simulink model "modechanger"  (R2022b)
settings: Solver=FixedStepAuto  StartTime=0.0  StopTime=inf  FixedStep=0.01  RelTol=1e-3
libraries: robotlib x7
settings Model: Creator=sprinkle  LastModifiedBy=sprinkle
settings SolverCC: AlgebraicLoopSolver=TrustRegion
settings OptimizationCC: UseFloatMulNetSlope=on  EnhancedBackFolding=on  EfficientFloat2IntCast=on  MaxStackSize=64  OptimizeBlockOrder=speed  DifferentSizesBufferReuse=on  OptimizationCustomize=off
settings DebuggingCC: ParameterTunabilityLossMsg=error  UnconnectedInputMsg=warning  UnconnectedOutputMsg=warning  UnconnectedLineMsg=warning  SFMachineParentedDataDiag=warning
settings HardwareCC: ProdBitPerPointer=32  ProdBitPerSizeT=32  ProdBitPerPtrDiffT=32  ProdLargestAtomicFloat=None  ProdIntDivRoundTo=Undefined  ProdEndianess=Unspecified  ProdWordSize=32  ProdHWDeviceType=Generic->Unspecified (assume 32-bit Generic)  UseEmbeddedCoderFeatures=off
settings ModelReferenceCC: EnableRefExpFcnMdlSchedulingChecks=on
settings SFSimCC: MATLABDynamicMemAlloc=off  SimTargetLang=C++
settings RTWCC: Description=Embedded Coder  SystemTargetFile=ert.tlc  HardwareBoard=Robot Operating System (ROS)  TLCOptions="-aInlineSetEventsForThisBaseRateFcn=TLC_FALSE -aSuppressMultiTaskScheduler=TLC_FALSE  -aRateBasedStepFcn=0"  TemplateMakefile=ert_default_tmf  GenerateReport=on  Toolchain=Catkin  BuildConfiguration=Faster Runs  LaunchReport=on  TargetLang=C++
settings CodeAppCC: ForceParamTrailComments=on  OperatorAnnotations=on
settings ERTTargetCC: ERTCustomFileBanners=off  SupportNonFinite=off  SupportContinuousTime=on  SupportNonInlinedSFcns=on  RemoveResetFunc=off  ModelStepFunctionPrototypeControlCompliant=off  RootIOFormat=Structure reference

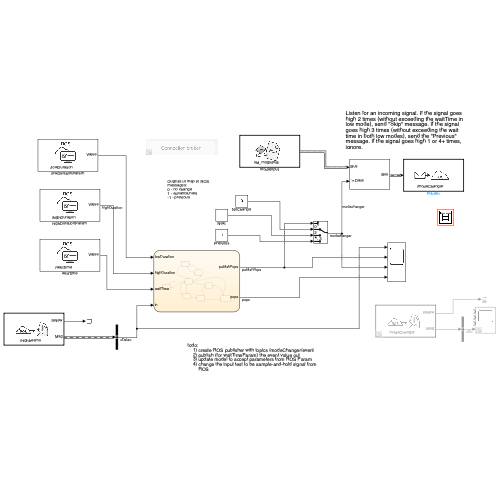
[thumbnail: Simulink's stored preview of the top-level diagram]
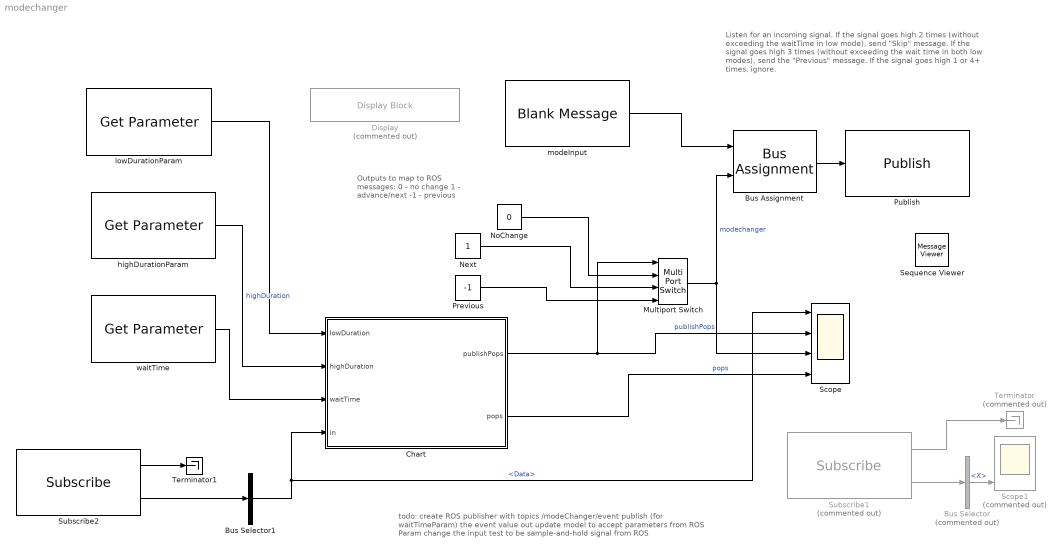
== system modechanger ==
  note: todo:
      | create ROS publisher with topics /modeChanger/event
      | publish (for waitTimeParam) the event value out
      | update model to accept parameters from ROS Param
      | change the input test to be sample-and-hold signal from ROS
  note: Listen for an incoming signal. If the signal goes high 2 times (without exceeding the waitTime in low mode), send "Skip" message. If the signal goes high 3 times (without exceeding the wait time in both low modes), send the "Previous" message. If the signal goes high 1 or 4+ times, ignore.
  note: Outputs to map to ROS messages:
      | 0 - no change
      | 1 - advance/next
      | -1 - previous
  Bus Assignment : BusAssignment  AssignedSignals=Data
  Bus Selector : BusSelector  Commented=on  DialogController=Simulink.DDGSource_BusSelector  OutputSignals=Linear.X
  Bus Selector1 : BusSelector  DialogController=Simulink.DDGSource_BusSelector  OutputSignals=Data
  Chart : Stateflow chart  TreatAsAtomicUnit=on
  Display : DisplayBlock  Commented=on  LabelPosition=Hide  Transparency=1
  Multiport Switch : MultiPortSwitch  DataPortOrder=Specify indices  DataPortIndices={0,2,3}  SaturateOnIntegerOverflow=off  InputSameDT=off
  Next : Constant  OutDataTypeStr=int8
  NoChange : Constant  Value=0  OutDataTypeStr=int8
  Previous : Constant  Value=-1  OutDataTypeStr=int8
  Publish : robotlib/Publish  topicSource=Specify your own  topic=/modeChanger  messageType=std_msgs/Int8  legacyBusStruct=off  messageQueueLength=1
      settings: LibrarySourceBlock=roslib/ROS/Publish
  Scope : Scope  NumInputPorts=4
  Scope1 : Scope  Commented=on  NumInputPorts=4
  Sequence Viewer : MessageViewer  History=1000  SavedRootId=#
  Subscribe1 : robotlib/Subscribe  Commented=on  topicSource=Specify your own  topic=modeChanger  messageType=geometry_msgs/Twist  SampleTime=0.05  legacyBusStruct=off  messageQueueLength=1
  Subscribe2 : robotlib/Subscribe  topicSource=Specify your own  topic=/highbeams  messageType=std_msgs/Float64  SampleTime=-1  legacyBusStruct=off  messageQueueLength=10
  Terminator : Terminator  Commented=on
  Terminator1 : Terminator
  highDurationParam : robotlib/Get Parameter  ParameterSource=Specify your own  ParameterName=/highDuration  ParameterType=double  ParameterMaxArrayLength=16  ParameterInitialValue=0.05  SampleTime=-1  ShowErrorCodeOutput=off  ModelName=modechanger  BlockId=ParamGet_modechanger_59
  lowDurationParam : robotlib/Get Parameter  ParameterSource=Specify your own  ParameterName=/lowDuration  ParameterType=double  ParameterMaxArrayLength=16  ParameterInitialValue=0.02  SampleTime=-1  ShowErrorCodeOutput=off  ModelName=modechanger  BlockId=ParamGet_modechanger_56
  modeInput : robotlib/Blank Message  messageClass=Message  entityType=std_msgs/Int8  messageType=std_msgs/Int8  SampleTime=-1  legacyBusStruct=off
  waitTime : robotlib/Get Parameter  ParameterSource=Specify your own  ParameterName=/waitTime  ParameterType=double  ParameterMaxArrayLength=16  ParameterInitialValue=0.3  SampleTime=-1  ShowErrorCodeOutput=off  ModelName=modechanger  BlockId=ParamGet_modechanger_60
  wires:
  highDurationParam/1 -> Chart/2(highDuration)  "highDuration"
  Subscribe2/2 -> Bus Selector1/1
  Previous/1 -> Multiport Switch/4
  Next/1 -> Multiport Switch/3
  Multiport Switch/1 -> Scope/3, Bus Assignment/2  "modechanger"
  NoChange/1 -> Multiport Switch/2
  Bus Assignment/1 -> Publish/1
  modeInput/1 -> Bus Assignment/1
  Subscribe1/1 -> Terminator/1
  Subscribe1/2 -> Bus Selector/1
  Bus Selector/1 -> Scope1/4  "<X>"
  Subscribe2/1 -> Terminator1/1
  Bus Selector1/1 -> Scope/1, Chart/4(in)  "<Data>"
  lowDurationParam/1 -> Chart/1(lowDuration)
  waitTime/1 -> Chart/3(waitTime)
  Chart/2(pops) -> Scope/4  "pops"
  Chart/1(publishPops) -> Multiport Switch/1, Scope/2  "publishPops"

== stateflow chart modechanger/Chart ==
  state ResetPops
    entry: pops=0;
  state Reset
  state idle
  state HeldIn
  state initialize
    entry: pops=0
  state High
  state Pop
    entry: pops=pops+1;
  state Debounce
  Reset -> ResetPops [order 2] : [pops<=1]
  ResetPops -> idle : after(waitTime,sec){publishPops=0;}
  Reset -> ResetPops [order 1] : [pops>1]{publishPops=pops;}
  idle -> Reset [order 2] : after(waitTime,sec)
  Pop -> idle [order 1] : [pops<=3]
  initialize -> idle
  (default) -> initialize
  HeldIn -> idle : [in==0]{pops=0;}
  High -> idle [order 1] : [in==0]
  idle -> High [order 1] : [in>0]{publishPops=0;}
  Pop -> HeldIn [order 2] : [pops>3]
  Debounce -> HeldIn [order 1] : after(waitTime,sec)
  High -> Debounce [order 2] : after(highDuration,sec)
  Debounce -> Pop [order 2] : [in==0]
  data: lowDuration input; highDuration input; waitTime input; in input; publishPops output int8; pops output int8
